simulink model "Second_order_system_CS"  (R2023b)
settings: Solver=VariableStepAuto  StartTime=0.0  StopTime=10.0  RelTol=1e-3
settings Model: Creator=devan  LastModifiedBy=devan

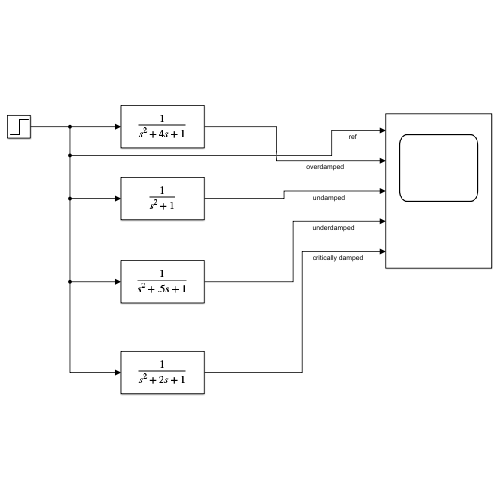
[thumbnail: Simulink's stored preview of the top-level diagram]
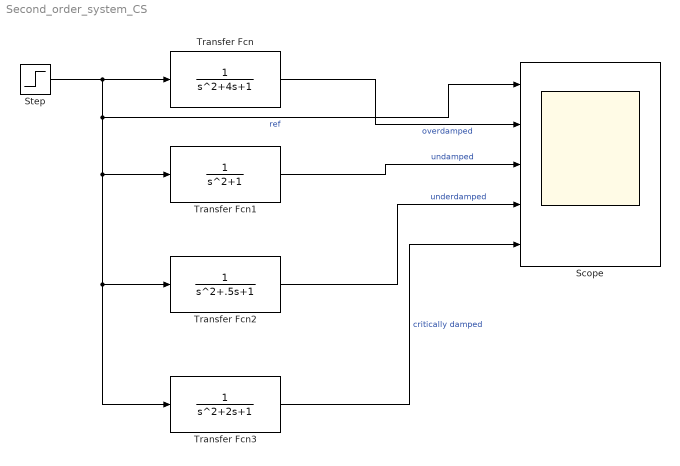
== system Second_order_system_CS ==
  Scope : Scope  NumInputPorts=5
  Step : Step  Time=0.1  SampleTime=0
  Transfer Fcn : TransferFcn  Denominator=[1 4 1]
  Transfer Fcn1 : TransferFcn  Denominator=[1 0 1]
  Transfer Fcn2 : TransferFcn  Denominator=[1 .5 1]
  Transfer Fcn3 : TransferFcn
  wires:
  Step/1 -> Transfer Fcn3/1, Transfer Fcn2/1, Transfer Fcn1/1, Scope/1, Transfer Fcn/1  "ref"
  Transfer Fcn/1 -> Scope/2  "overdamped"
  Transfer Fcn1/1 -> Scope/3  "undamped"
  Transfer Fcn2/1 -> Scope/4  "underdamped"
  Transfer Fcn3/1 -> Scope/5  "critically damped"
